simulink library "sun_sensor_lib"  (R2016b)
settings: Solver=VariableStepAuto  StartTime=0.0  StopTime=10.0  RelTol=1e-3
libraries: dspmathops x2, vrlib x1, aerolibutil x1, aerolibtransform2 x1
settings Model: Creator=Taylor  LastModifiedBy=Taylor
settings OptimizationCC: LifeSpan=inf
settings DebuggingCC: SFExecutionAtInitializationDiag=none

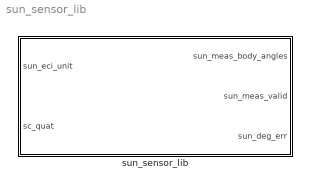
== system sun_sensor_lib ==
  "sun_sensor_lib " : Subsystem

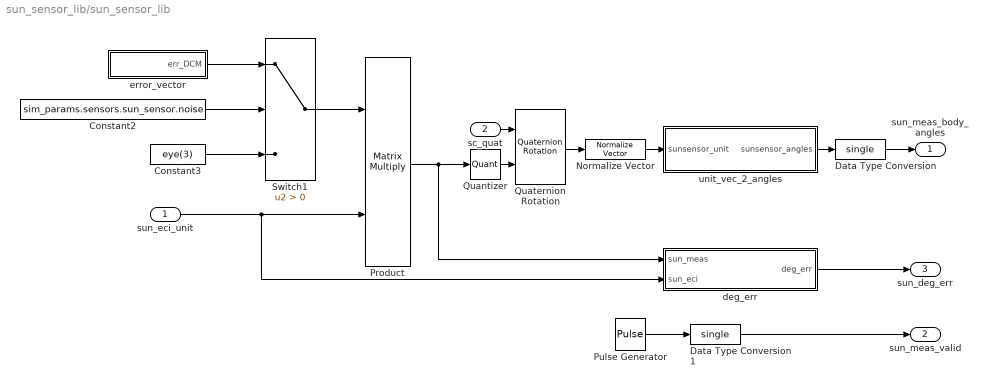
== system sun_sensor_lib/sun_sensor_lib  ==
  sun_eci_unit : Inport
  sc_quat : Inport  Port=2
  Constant2 : Constant  Value=sim_params.sensors.sun_sensor.noise
  Constant3 : Constant  Value=eye(3)
  Data Type Conversion : DataTypeConversion  OutDataTypeStr=single
  Data Type Conversion1 : DataTypeConversion  OutDataTypeStr=single
  Normalize Vector : vrlib/Utilities/Normalize Vector  maxzero=0
  Product : Product  Multiplication=Matrix(*)  RndMeth=Zero
  Pulse Generator : DiscretePulseGenerator  PulseType=Time based  Period=10  PulseWidth=sim_params.sensors.sun_sensor.valid_pct
  Quantizer : Quantizer  QuantizationInterval=sim_params.sensors.sun_sensor.resolution
  Quaternion Rotation : aerolibutil/Quaternion Rotation
  Switch1 : Switch  Criteria=u2 > Threshold
  deg_err : Subsystem
  error_vector : Subsystem
  unit_vec_2_angles : Subsystem
  sun_meas_body_angles : Outport
  sun_meas_valid : Outport  Port=2
  sun_deg_err : Outport  Port=3
  wires:
  sc_quat/1 -> Quaternion Rotation/1
  Pulse Generator/1 -> Data Type Conversion1/1
  Constant2/1 -> Switch1/2
  Constant3/1 -> Switch1/3
  Switch1/1 -> Product/1
  sun_eci_unit/1 -> deg_err/2(sun_eci), Product/2
  Product/1 -> deg_err/1(sun_meas), Quantizer/1
  Quantizer/1 -> Quaternion Rotation/2
  deg_err/1(deg_err) -> sun_deg_err/1
  Data Type Conversion1/1 -> sun_meas_valid/1
  error_vector/1(err_DCM) -> Switch1/1
  Quaternion Rotation/1 -> Normalize Vector/1
  Data Type Conversion/1 -> sun_meas_body_angles/1
  unit_vec_2_angles/1(sunsensor_angles) -> Data Type Conversion/1
  Normalize Vector/1 -> unit_vec_2_angles/1(sunsensor_unit)

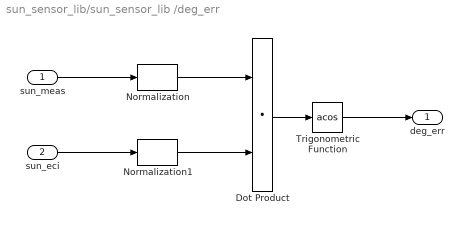
== system sun_sensor_lib/sun_sensor_lib /deg_err ==
  sun_meas : Inport
  sun_eci : Inport  Port=2
  Dot Product : DotProduct  InputSameDT=on  OutDataTypeStr=Inherit: Inherit via internal rule
  Normalization : dspmathops/Normalization  NormType=2-norm  Bias=1e-10  NormOver=Each column  Dimension=1  outputDataTypeStr=Inherit: Same as product output  outputLastDataTypeStr=Inherit: Same as product output  outputMin=[]  outputMax=[]  accumDataTypeStr=Inherit: Same as product output  accumLastDataTypeStr=Inherit: Same as product output  roundingMode=Floor  overflowMode=off
  Normalization1 : dspmathops/Normalization  NormType=2-norm  Bias=1e-10  NormOver=Each column  Dimension=1  outputDataTypeStr=Inherit: Same as product output  outputLastDataTypeStr=Inherit: Same as product output  outputMin=[]  outputMax=[]  accumDataTypeStr=Inherit: Same as product output  accumLastDataTypeStr=Inherit: Same as product output  roundingMode=Floor  overflowMode=off
  Trigonometric Function : Trigonometry  Operator=acos
  deg_err : Outport
  wires:
  sun_meas/1 -> Normalization/1
  Normalization/1 -> Dot Product/1
  sun_eci/1 -> Normalization1/1
  Dot Product/1 -> Trigonometric Function/1
  Trigonometric Function/1 -> deg_err/1
  Normalization1/1 -> Dot Product/2

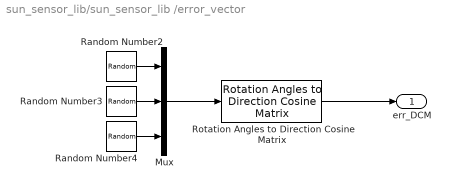
== system sun_sensor_lib/sun_sensor_lib /error_vector ==
  Mux : Mux  Inputs=3
  Random Number2 : RandomNumber  Variance=sim_params.sensors.sun_sensor.varx  SampleTime=sim_params.sensors.sun_sensor.sample_time_s
  Random Number3 : RandomNumber  Variance=sim_params.sensors.sun_sensor.vary  Seed=1  SampleTime=sim_params.sensors.sun_sensor.sample_time_s
  Random Number4 : RandomNumber  Variance=sim_params.sensors.sun_sensor.varz  Seed=2  SampleTime=sim_params.sensors.sun_sensor.sample_time_s
  Rotation Angles to Direction Cosine Matrix : aerolibtransform2/Rotation Angles to Direction Cosine Matrix  rotationOrder=ZYX
  err_DCM : Outport
  wires:
  Rotation Angles to Direction Cosine Matrix/1 -> err_DCM/1
  Mux/1 -> Rotation Angles to Direction Cosine Matrix/1
  Random Number3/1 -> Mux/2
  Random Number2/1 -> Mux/1
  Random Number4/1 -> Mux/3

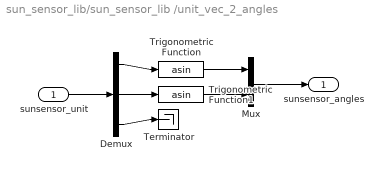
== system sun_sensor_lib/sun_sensor_lib /unit_vec_2_angles ==
  sunsensor_unit : Inport
  Demux : Demux  Outputs=3
  Mux : Mux  Inputs=2
  Terminator : Terminator
  Trigonometric Function : Trigonometry  Operator=asin
  Trigonometric Function1 : Trigonometry  Operator=asin
  sunsensor_angles : Outport
  wires:
  sunsensor_unit/1 -> Demux/1
  Demux/1 -> Trigonometric Function/1
  Demux/2 -> Trigonometric Function1/1
  Trigonometric Function/1 -> Mux/1
  Trigonometric Function1/1 -> Mux/2
  Mux/1 -> sunsensor_angles/1
  Demux/3 -> Terminator/1
